simulink model "Q3"  (R2015b)
settings: Solver=ode1  StartTime=0.0  StopTime=3.14  FixedStep=0.002  MaxStep=.1  RelTol=1e-3
PreLoadFcn:
  | load_inputs
values from neighbouring files (symbols this model uses):
  r = 0.012    [Q2biv.m]    (also in Q4c.m = 0.03 * (     sin(pi*x/d)     + (1/3)*sin(3*pi*x/d)     + (1/; load_inputs.m = 0.05)
  v_L = w*(r_P-(L/2))    (= 0.95)    [load_inputs.m]
  v_P = 1    [load_inputs.m]
  v_R = w*(r_P+(L/2))    (= 1.05)    [load_inputs.m]
  w_L = v_L/r    (= 19)    [load_inputs.m]
  w_R = v_R/r    (= 21)    [load_inputs.m]
settings Model: Creator=The MathWorks, Inc.  LastModifiedBy=SooJengTan
settings DataIOCC: SaveFormat=Array
settings OptimizationCC: ExpressionDepthLimit=2147483647
settings DebuggingCC: UnderspecifiedInitializationDetection=Classic  MergeDetectMultiDrivingBlocksExec=none  SolverPrmCheckMsg=warning  FcnCallInpInsideContextMsg=UseLocalSettings  StateNameClashWarn=warning
settings HardwareCC: ProdBitPerPointer=32  ProdLargestAtomicFloat=None  ProdIntDivRoundTo=Undefined  ProdEndianess=Unspecified  ProdWordSize=32  ProdHWDeviceType=32-bit Generic
settings GRTTargetCC: GeneratePreprocessorConditionals=Disable all  CombineOutputUpdateFcns=off  GRTInterface=on
settings ConfigComp: CovModelRefEnable=Off

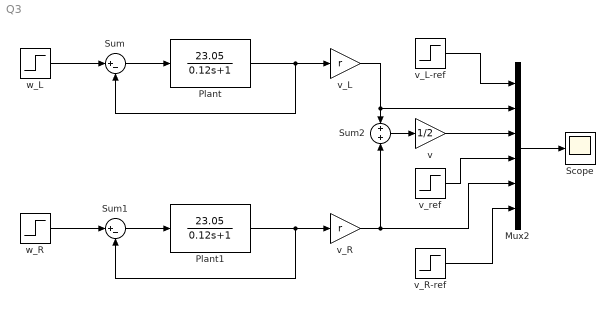
== system Q3 ==
  Mux2 : Mux  Inputs=6
  Plant : TransferFcn  Numerator=[23.05]  Denominator=[0.12 1]
  Plant1 : TransferFcn  Numerator=[23.05]  Denominator=[0.12 1]
  Scope : Scope
  Sum : Sum  Inputs=|+-
  Sum1 : Sum  Inputs=|+-
  Sum2 : Sum  Inputs=+|+
  v : Gain  Gain=1/2
  v_L : Gain  Gain=r
  v_L-ref : Step  Time=0  After=v_L  SampleTime=0
  v_R : Gain  Gain=r
  v_R-ref : Step  Time=0  After=v_R  SampleTime=0
  v_ref : Step  Time=0  After=v_P  SampleTime=0
  w_L : Step  Time=0  After=w_L  SampleTime=0
  w_R : Step  Time=0  After=w_R  SampleTime=0
  wires:
  w_L/1 -> Sum/1
  Sum/1 -> Plant/1
  Plant/1 -> Sum/2, v_L/1
  w_R/1 -> Sum1/1
  Sum1/1 -> Plant1/1
  Plant1/1 -> v_R/1, Sum1/2
  v_R/1 -> Mux2/5, Sum2/2
  v_L/1 -> Mux2/2, Sum2/1
  Sum2/1 -> v/1
  v/1 -> Mux2/3
  v_ref/1 -> Mux2/4
  Mux2/1 -> Scope/1
  v_R-ref/1 -> Mux2/6
  v_L-ref/1 -> Mux2/1
